simulink model "control_pinyu"  (R2025a)
settings: Solver=VariableStepAuto  StartTime=0.0  StopTime=10.0  RelTol=1e-3
undefined symbols (not defined in the file or in its folder): R, Z
settings Model: Creator=Administrator  LastModifiedBy=Administrator

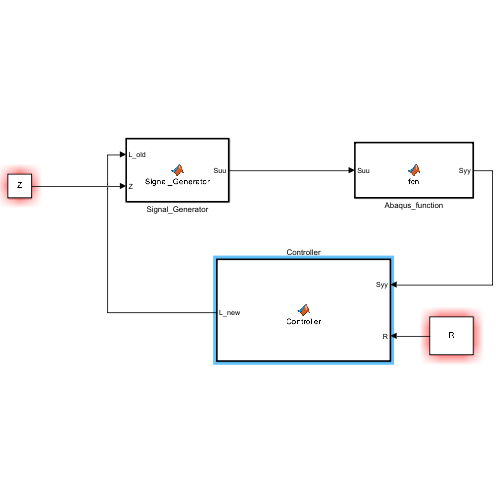
[thumbnail: Simulink's stored preview of the top-level diagram]
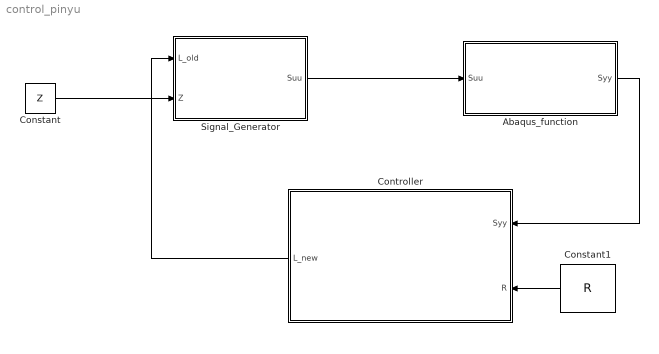
== system control_pinyu ==
  Abaqus_function : MATLAB Function  TreatAsAtomicUnit=on
  Constant : Constant  Value=Z
  Constant1 : Constant  Value=R
  Controller : MATLAB Function  TreatAsAtomicUnit=on
  Signal_Generator : MATLAB Function  TreatAsAtomicUnit=on
  wires:
  Constant/1 -> Signal_Generator/2(Z)
  Controller/1(L_new) -> Signal_Generator/1(L_old)
  Signal_Generator/1(Suu) -> Abaqus_function/1(Suu)
  Abaqus_function/1(Syy) -> Controller/1(Syy)
  Constant1/1 -> Controller/2(R)

== matlab function control_pinyu/Controller ==
  data: Syy input; R input; L_new output
function L_new = Controller( Syy, R)
% Controller
% 功能：基于矩阵幂次算法更新控制变量
% 配置：1Hz分辨率 (N_half=2561)
% 输入：
%   L_old:    [2561x2x2] 上一时刻的控制变量
%   Syy:      [2561x2x2] 平均响应谱 (Response Spectrum)
%   R:        [2561x2x2] 参考谱 (Reference Spectrum)

    % %% 1. 参数设置
    % 收敛因子 (Convergence Factor)
    epsilon = 0.5; 
    
    % % 【新增】收敛监控变量
    % persistent iteration_count convergence_history
    % if isempty(iteration_count)
    %     iteration_count = 0;
    %     convergence_history = [];
    % end
    % 正定性保护阈值 (Regularization)
    reg_val = 1e-12; 
    
    % %% 2. 逻辑判断
    if isPeriod
         % iteration_count = iteration_count + 1;
        % === 触发修正 ===
        % 【新增】检查 Syy 是否有效 (非零矩阵)
      % Syy_max = max(abs(Syy(:)));
       
       % if Syy_max < 1e-20
       %  % Syy 无效 (全零或接近零)，跳过本次修正
       %  L_new = L_old;
       %  return;  % 提前返回
       % end
       
       % 修改后
       Syy_max = max(abs(Syy(:)));
       % 【新增】NaN/Inf 保护
       if ~isfinite(Syy_max) || Syy_max < 1e-20
        % Syy 无效 (全零、NaN或Inf)，跳过本次修正
        L_new = L_old;
        return;
      end
        % 初始化输出矩阵
        % 必须显式声明为复数，防止后续计算产生虚部时报错
        L_new = complex(zeros(size(L_old)));
        N_half = size(L_old, 1);
        % 【新增】收敛误差计算
        %total_error = 0;
        
        for k = 1:N_half
            % 提取当前频点的矩阵 (2x2)
            R_k = squeeze(R(k, :, :));
            Syy_k = squeeze(Syy(k, :, :));
            L_old_k = squeeze(L_old(k, :, :));
           % 【新增】频点级别 NaN/Inf 保护
            if any(~isfinite(Syy_k(:))) || any(~isfinite(R_k(:))) || any(~isfinite(L_old_k(:)))
                L_new(k, :, :) = L_old_k;
                continue;
            end

            
            % --- 步骤 A: 响应谱 Syy 分解 (Ls) ---
            % 保护机制：确保 Syy 正定，替代 try-catch
            % 1. 强制对称
            Syy_k = (Syy_k + Syy_k') / 2;
            % 2. 特征值分解
            [V, D] = eig(Syy_k);
            d_diag = diag(D);
            % 3. 如果特征值太小或为负，强制拉高
            if any(d_diag <= reg_val)
                d_diag = max(d_diag, reg_val);
                Syy_k = V * diag(d_diag) * V';
            end
            
            % Cholesky 分解: Syy = Ls * Ls'
            Ls = chol(Syy_k, 'lower');
            
            % --- 步骤 B: 参考谱 R 分解 (Lr) ---
            % 同样进行保护，尽管 R 通常是正定的
            R_k = (R_k + R_k') / 2;
            [Vr, Dr] = eig(R_k);
            dr_diag = diag(Dr);
            if any(dr_diag <= reg_val)
                 dr_diag = max(dr_diag, reg_val);
                 R_k = Vr * diag(dr_diag) * Vr';
            end
            Lr = chol(R_k, 'lower');
            
            % --- 步骤 C: 计算误差矩阵 Delta ---
            % Delta = Lr * inv(Ls)
            % 使用右除 / 提高精度 (相当于 * inv(Ls))
            Delta = Lr / Ls;
            
           % 【新增】Delta 条件数检查
           if rcond(Delta) < 1e-10
               % Delta 接近奇异，跳过本频点修正
               L_new(k, :, :) = L_old_k;
               continue;
           end

            % --- 步骤 D: 矩阵幂次修正 ---
            % Correction = Delta ^ epsilon
            % MATLAB Function 支持矩阵幂运算 '^'
            Correction = Delta ^ epsilon;
            
            % --- 步骤 E: 更新控制变量 ---
            % L_new = Correction * L_old
            L_new(k, :, :) = Correction * L_old_k;

            % 【新增】累加误差
            %total_error = total_error + norm(Syy_k - R_k, 'fro');
        end
        % 【新增】记录收敛历史（可选：通过输出端口导出）
        %avg_error = total_error / N_half;
        %fprintf('Iteration %d: Avg Error = %.6e\n', iteration_count, avg_error);
        
    else
        % === 非触发时刻，保持输出 ===
        L_new = L_old;
    end
    
end

== matlab function control_pinyu/Signal_Generator ==
  data: L_old input; Suu output; Z input

function Suu = Signal_Generator(L_old, Z)
% Signal_Generator
% 功能：基于矩阵幂次控制变量 L_old，生成 MIMO 时域驱动力信号
% 方法：频域高斯随机化 + IFFT + 重叠相加 (Overlap-Add)
% 配置：1Hz分辨率 (N=5120, N_half=2561)
% 输入：
%   L_old: [2561x2x2] 加速度域控制因子 (复数下三角)
%   Z:     [2561x2x2] 逆系统矩阵 (Force/Acceleration)

    % %% 1. 参数定义
    N = 5120;               % FFT 点数 (1Hz分辨率)
    Overlap = 2560;         % 重叠点数 (50%)
    Fs = 5120;              % 采样率
    df = Fs / N;            % 频率分辨率
    N_half = N/2 + 1;       % 2561
    
    % %% 2. 持久变量 (用于连续播放)
    persistent Play_Buffer    % 当前播放缓冲区 [512 x 2]
    persistent Overlap_Buffer % 重叠缓冲区 [512 x 2] (存储上一帧的尾部)
    persistent play_idx       % 播放指针 (1 ~ 512)
    persistent h_win          % 汉宁窗
    
    % 初始化
    if isempty(play_idx)
        play_idx = Overlap + 1;
        Play_Buffer = zeros(Overlap, 2);
        Overlap_Buffer = zeros(Overlap, 2);
        
        % 预计算汉宁窗 (1024x1)
        % 注意：合成时通常使用 "Periodic" 窗或标准窗，这里用标准汉宁窗
        %h_win = 0.5 * (1 - cos(2 * pi * (0:N-1)' / (N-1)));
        % 修改后 (周期性Hann窗，满足50% overlap COLA条件)
        h_win = 0.5 * (1 - cos(2 * pi * (0:N-1)' / N));
    end
    
    % %% 3. 检查缓冲区状态
    % 如果当前缓冲区播放完毕 (play_idx > 512)，则生成新的一帧
    if play_idx > Overlap
        
        % === A. 频域合成 ===
        % 初始化全频段谱 (双边谱) [1024 x 2]
        U_full = complex(zeros(N, 2));
        
        % 缩放因子：将 PSD (unit^2/Hz) 转换为 FFT 幅值
        % 理论推导：S = |U|^2 * dt / N  => |U| ~ sqrt(S * N * Fs) ... 
        % 工程近似：sqrt(df) 用于积分，N 用于 IFFT 增益
        % 这里使用简化的能量匹配系数，具体数值可能需要根据 Response_spectrum 模块的 scale_factor 微调
        % 这里的 sqrt(df/2) 是将单边 PSD 密度转换为单边 rms 幅值 (除以2是因为双边)
        %Gen_Gain = sqrt(df/2) * N; 

        % 【修复】与 Response_spectrum_calculation 的 scale_factor 完全对称
       % 分析模块: scale_factor = 2 / (Fs * W_factor)
       % 生成模块: Gen_Gain 需要满足 |IFFT(U)|^2 的期望 = 目标PSD * df
        %
% 推导:
%   分析时: S = |Y|^2 * 2 / (Fs * W_factor)
%   生成时: 我们要 E[|u(t)|^2] = S_target * df
%          而 u(t) = IFFT(U), 所以 E[sum(|u|^2)] = E[|U|^2] / N
%          因此 |U_k|^2 = S_target * Fs * W_factor / 2 * N / N = S_target * Fs * W_factor / 2
%          所以 |U_k| = sqrt(S_target) * sqrt(Fs * W_factor / 2)
%
% 由于 S_target = |L|^2 (L 已包含振幅信息)，所以:
W_factor = sum(h_win.^2);  % 汉宁窗能量因子 ≈ 512 for N=1024
Gen_Gain = sqrt(Fs * W_factor / 2);  % ≈ sqrt(5120 * 512 / 2) ≈ 1144.55
        
        % 循环计算单边谱 (DC ~ Nyquist)
        for k = 1:N_half
            
            % 1. 提取矩阵
            L_k = squeeze(L_old(k, :, :)); % [2x2]
            Z_k = squeeze(Z(k, :, :));     % [2x2]
            
            % 2. 计算驱动因子 D = Z * L (Force Domain)
            D_k = Z_k * L_k;               % [2x2]
            
            % 3. 生成独立复高斯白噪声向量 w ~ CN(0, I)
            % 实部虚部各为 N(0, 0.5)，保证模的期望为 1
            w = (randn(2, 1) + 1j * randn(2, 1)) / sqrt(2);
            
            % 4. 合成驱动谱 U = D * w
            U_k = D_k * w;                 % [2x1]
            
            % 5. 存入全频谱 (正频率)
            U_full(k, :) = U_k.' * Gen_Gain;
        end
        
       % 修改前
        % === B. 构造 Hermitian 对称 (保证时域为实数) ===
        % DC(1) 和 Nyquist(513) 虚部置 0
        %U_full(1, :) = real(U_full(1, :));
        %%U_full(N_half, :) = real(U_full(N_half, :));

       % 修改后 (补偿DC/Nyquist的方差减半问题)
        % === B. 构造 Hermitian 对称 (保证时域为实数) ===
        % DC(1) 和 Nyquist(2561) 使用实高斯，并补偿方差 (乘sqrt(2))
        U_full(1, :) = real(U_full(1, :)) * sqrt(2);
        U_full(N_half, :) = real(U_full(N_half, :)) * sqrt(2);
        
        % 填充负频率 (514 ~ 1024) = conj(flip(2 ~ 512))
        U_full(N_half+1 : N, :) = conj(flipud(U_full(2 : N_half-1, :)));
        
        % === C. IFFT 与 加窗 ===
        u_time_block = ifft(U_full, N, 1, 'symmetric'); % [1024 x 2] (实数)
        
        % 加窗 (Element-wise)
        u_win = u_time_block .* h_win;
        
        % === D. 重叠相加 (Overlap-Add) ===
        % 前 512 点：与上一帧的尾部叠加 -> 放入播放缓冲区
        Play_Buffer = u_win(1:Overlap, :) + Overlap_Buffer;
        
        % 后 512 点：存入重叠缓冲区，等待下一帧
        Overlap_Buffer = u_win(Overlap+1:N, :);
        
        % 重置播放指针
        play_idx = 1;
    end
    
    % %% 4. 输出当前采样点
      u = Play_Buffer(play_idx, :).'; 
    
    % 更新指针
    play_idx = play_idx + 1;

end

== matlab function control_pinyu/Abaqus_function ==
  data: Suu input; Syy output
function Syy = fcn(Suu)
